simulink library "GASSTAGES_WD_MASTER"  (Simulink 8.5)
settings: Solver=ode45  StartTime=0.0  StopTime=10.0  RelTol=1e-3
libraries: cdsFilt x1, cdsRms x1, cdsTP x1, cdsEpicsOut x1, cdsEpicsIn x1
settings Model: Creator=controls  LastModifiedBy=controls

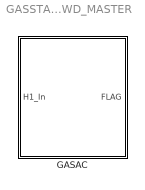
== system GASSTAGES_WD_MASTER ==
  GASAC : Subsystem

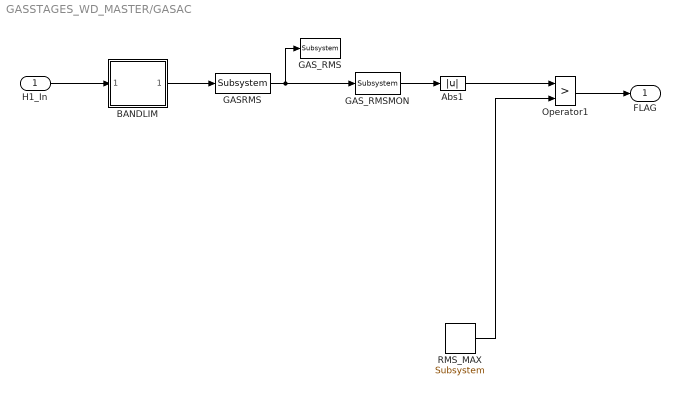
== system GASSTAGES_WD_MASTER/GASAC ==
  H1_In : Inport
  Abs1 : Abs
  BANDLIM : Subsystem
  GASRMS : cdsRms/Subsystem  Tag=cdsRms  Description=|
      | Purpose:
      | Calculate an RMS based on the input signal.
      settings: AttributesFormatString=%<Tag>
  GAS_RMS : cdsTP/Subsystem  Tag=Test Point
      settings: AttributesFormatString=%<Tag>
  GAS_RMSMON : cdsEpicsOut/Subsystem  Tag=cdsEpicsOutput  Description=|
      | Purpose:                                          
      | Output a FE signal to an EPICS channel.           
      |                                                   
      | Operation:                                        
      | Takes input value and passes it to EPICS record.  
      |                                                   
      | Usage:                                            
      | Name the part with the desired EPICS rrecord name.
      settings: AttributesFormatString=%<Tag>
  Operator1 : RelationalOperator  Operator=>  OutDataTypeStr=boolean
  RMS_MAX : cdsEpicsIn/Subsystem  Tag=cdsEpicsIn  Description=|
      | Purpose:                                                                              
      | Create an EPICS input channel connection to the FE realtime controls.                 
      |                                                                                       
      | Operation:                                                                            
      | Outputs value from an EPICS ai record. Value is floating point with a precision of 3..
      |                                                                                       
      | Usage:                                                                                
      | Name the part with the desired EPICS channel name.
      settings: AttributesFormatString=%<Tag>
  FLAG : Outport
  wires:
  Operator1/1 -> FLAG/1
  GASRMS/1 -> GAS_RMSMON/1, GAS_RMS/1
  RMS_MAX/1 -> Operator1/2
  Abs1/1 -> Operator1/1
  GAS_RMSMON/1 -> Abs1/1
  H1_In/1 -> BANDLIM/1(H1_In)
  BANDLIM/1(H1_Out) -> GASRMS/1

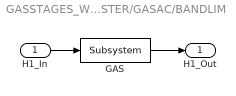
== system GASSTAGES_WD_MASTER/GASAC/BANDLIM ==
  H1_In : Inport
  GAS : cdsFilt/Subsystem  Tag=cdsFilt  Description=|
      | Purpose:                                                                                                                                                                                                                                  
      | Standard CDS IIR filter module.                                                                                                                                                                                                           
      |                                                                                                                                                                                                                                           
      | Operation:                                                                                                                                                                                                                                
      | Consists of 10 second order section IIR filters, plus a ramped gain stage. In FE code, also provides pre-defined test points and excitation channel inputs. The filter coefficients are defined in the LIGO system using the 'foton' tool.
      |                                                                                                                                                                                                                                           
      | Usage:                                                                                                                                                                                                                                    
      | Name the part with the desired filter module name.
      settings: AttributesFormatString=%<Tag>
  H1_Out : Outport
  wires:
  GAS/1 -> H1_Out/1
  H1_In/1 -> GAS/1
